simulink model "part1"  (R2021b)
settings: Solver=VariableStepAuto  StartTime=0.0  StopTime=t_set  MaxStep=dt  RelTol=1e-3
model workspace (MAT data in the model file):
  Amp = 1
values from neighbouring files (symbols this model uses):
  E = Vc(2)    [CurrentVelocities.m]
  Kd = [kd_surge kd_sway kd_yaw]    [CurrentVelocities.m]    (also in Init.m = [7e6 7e6 1e9])
  Ki = [ki_surge ki_sway ki_yaw]    [CurrentVelocities.m]    (also in Init.m = [3e6 3e6 1e6])
  Kp = [kp_surge kp_sway kp_yaw]    [CurrentVelocities.m]    (also in Init.m = [4e7 4e7 2e8])
  N = Vc(1)    [CurrentVelocities.m]
  set_x = 10    [CurrentVelocities.m]
  set_y = 10    [CurrentVelocities.m]
  set_yaw = 0.785    [CurrentVelocities.m]
  vessel =     [matlab.mat]
undefined symbols (not defined in the file or in its folder): Hoerner
libraries: marine_hydro x1
settings Model: Creator=jonbjor  LastModifiedBy=petterhangerhagen
settings SolverCC: AlgebraicLoopSolver=TrustRegion
settings DataIOCC: ReturnWorkspaceOutputs=off
settings DebuggingCC: SFMachineParentedDataDiag=warning  ArithmeticOperatorsInVariantConditions=warning
settings SFSimCC: SimUseLocalCustomCode=off  CustomCodeUndefinedFunction=UseInterfaceOnly
settings RTWCC: RTWUseLocalCustomCode=off

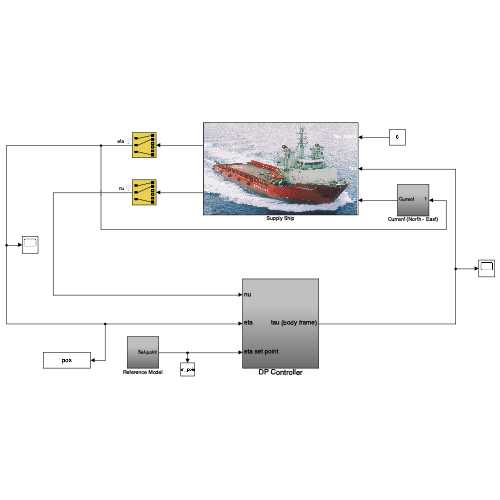
[thumbnail: Simulink's stored preview of the top-level diagram]
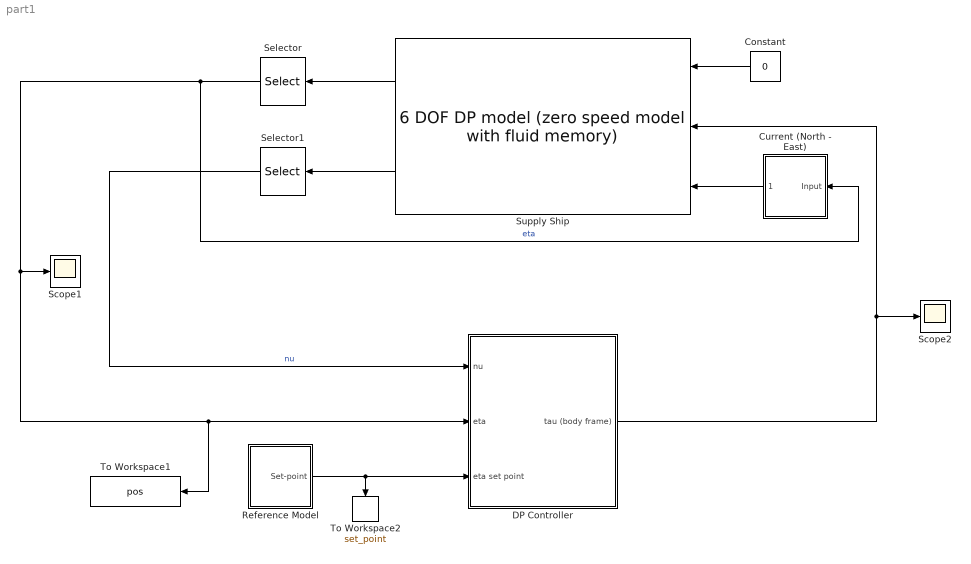
== system part1 ==
  Constant : Constant  Value=0
  Current (North - East) : Subsystem
  DP Controller : Subsystem
  Reference Model : Subsystem
  Scope1 : Scope
  Scope2 : Scope
  Selector : Selector  InputPortWidth=6  IndexOptions=Index vector (dialog)  Indices=[1 2 6]  OutputSizes=1
  Selector1 : Selector  InputPortWidth=6  IndexOptions=Index vector (dialog)  Indices=[1 2 6]  OutputSizes=1
  Supply Ship : marine_hydro/Hydro Library/6 DOF DP model  (zero speed model with fluid memory)  ABC=vesselABC  rho=1025  Axc=0.9*vessel.main.T*vessel.main.B  Ayc=0.9*vessel.main.T*vessel.main.Lpp  CX=1  CY_2D=Hoerner(vessel.main.B,vessel.main.T)  Bv=vessel.Bv  mask(6 DOF zero speed model){}
      link override "Integrator1 ": InitialCondition=nu0
      link override Integrator2: InitialCondition=eta0
      settings: SourceProductName=MSS Hydro
      mask Display:
      | image('supply.jpg');
      | color('white'); port_label('output', 1, 'eta')
      | color('white'); port_label('output', 2, 'nu')
      | color('white'); port_label('input', 1, 'tau_wave')
      | color('white'); port_label('input', 2, 'tau')
      | color('white'); port_label('input', 3, 'nu_c')
  To Workspace1 : ToWorkspace  VariableName=pos  SaveFormat=Timeseries  SampleTime=-1
  To Workspace2 : ToWorkspace  VariableName=set_point  SaveFormat=Timeseries  SampleTime=-1
  wires:
  Current (North - East)/1(Current) -> Supply Ship/3
  DP Controller/1(tau (body frame)) -> Scope2/1, Supply Ship/2
  Supply Ship/1 -> Selector/1
  Supply Ship/2 -> Selector1/1
  Selector/1 -> Current (North - East)/1(Input), Scope1/1, To Workspace1/1, DP Controller/2(eta)  "eta"
  Selector1/1 -> DP Controller/1(nu)  "nu"
  Constant/1 -> Supply Ship/1
  Reference Model/1(Set-point) -> To Workspace2/1, DP Controller/3(eta set point)

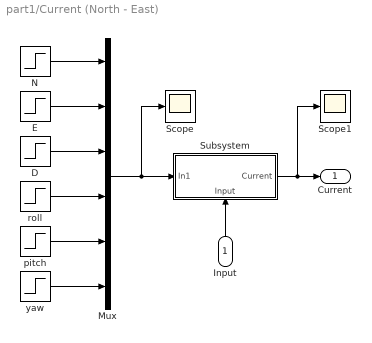
== system part1/Current (North - East) ==
  Input : Inport
  D : Step  Time=0  After=0  SampleTime=0
  E : Step  Time=0  After=E  SampleTime=0
  Mux : Mux  Inputs=6
  N : Step  Time=0  After=N  SampleTime=0
  Scope : Scope
  Scope1 : Scope
  Subsystem : Subsystem
      settings: PortSchema="{\"entries\":[{\"content\":{\"sides\":[{\"content\":{\"connectorIds\":[\"In1\"]},\"type\":\"ConnectorPlacement.EquallySpacedRectSide\",\"uuid\":\"4d23d725-1b89-4977-94a9-3d97af601562\"},{\"content\":{\"connectorIds\":[\"Out1\"],\"side\":\"RIGHT\"},\"type\":\"ConnectorPlacement.EquallySpacedRectSide\",\"uuid\":\"94064928-05d0-478d-b52c-d2c8e4fe82f6\"},{\"content\":{\"connectorIds\":[],\"side\":\"TOP\"},\"type\":\"ConnectorPlacement.EquallySpacedRectSide\",\"uuid\":\"63d93692-235d-465a-b22d-7c64b02cee26\"},{\"content\":{\"connectorIds\":[\"In2\"],\"side\":\"BOTTOM\"},\"type\":\"ConnectorPlacement.EquallySpacedRectSide\",\"uuid\":\"06906032-5717-4b79-be44-ac1ec3d34a3d\"}]},\"type\":\"ConnectorPlacement.EquallySpacedConnector\",\"uuid\":\"ca7e06dd-65f9-4f1a-a07c-a11377be80e1\"}],\"packageUris\":[\"http://schema.mathworks.com/mf0/Connector/R2020b\"],\"version\":\"1.0\"}"
  pitch : Step  Time=0  After=0  SampleTime=0
  roll : Step  Time=0  After=0  SampleTime=0
  yaw : Step  Time=0  After=0  SampleTime=0
  Current : Outport  VectorParamsAs1DForOutWhenUnconnected=off
  wires:
  N/1 -> Mux/1
  E/1 -> Mux/2
  Mux/1 -> Subsystem/1(In1), Scope/1
  D/1 -> Mux/3
  roll/1 -> Mux/4
  pitch/1 -> Mux/5
  yaw/1 -> Mux/6
  Input/1 -> Subsystem/2(Input)
  Subsystem/1(Current) -> Scope1/1, Current/1

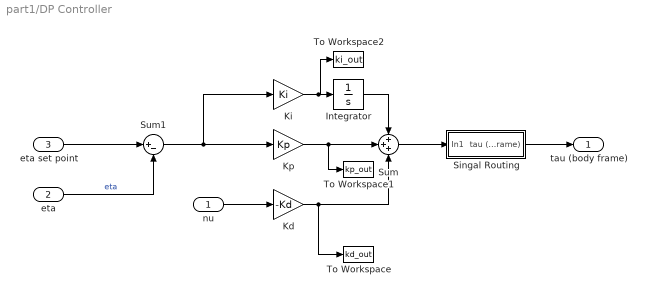
== system part1/DP Controller ==
  nu : Inport
  eta : Inport  Port=2
  eta set point : Inport  Port=3
  Integrator : Integrator
  Kd : Gain  Gain=-Kd
  Ki : Gain  Gain=Ki
  Kp : Gain  Gain=Kp
  Singal Routing : Subsystem
  Sum : Sum  Inputs=+++
  Sum1 : Sum  Inputs=|+-
  To Workspace : ToWorkspace  VariableName=kd_out  SaveFormat=Timeseries  SampleTime=-1
  To Workspace1 : ToWorkspace  VariableName=kp_out  SaveFormat=Timeseries  SampleTime=-1
  To Workspace2 : ToWorkspace  VariableName=ki_out  SaveFormat=Timeseries  SampleTime=-1
  tau (body frame) : Outport  VectorParamsAs1DForOutWhenUnconnected=off
  wires:
  Sum1/1 -> Ki/1, Kp/1
  eta set point/1 -> Sum1/1
  eta/1 -> Sum1/2  "eta"
  Kp/1 -> To Workspace1/1, Sum/2
  Ki/1 -> To Workspace2/1, Integrator/1
  Integrator/1 -> Sum/1
  Sum/1 -> Singal Routing/1(In1)
  Singal Routing/1(tau (body frame)) -> tau (body frame)/1
  Kd/1 -> Sum/3, To Workspace/1
  nu/1 -> Kd/1

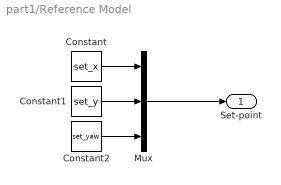
== system part1/Reference Model ==
  Constant : Constant  Value=set_x
  Constant1 : Constant  Value=set_y
  Constant2 : Constant  Value=set_yaw
  Mux : Mux  Inputs=3
  Set-point : Outport  VectorParamsAs1DForOutWhenUnconnected=off
  wires:
  Mux/1 -> Set-point/1
  Constant/1 -> Mux/1
  Constant1/1 -> Mux/2
  Constant2/1 -> Mux/3

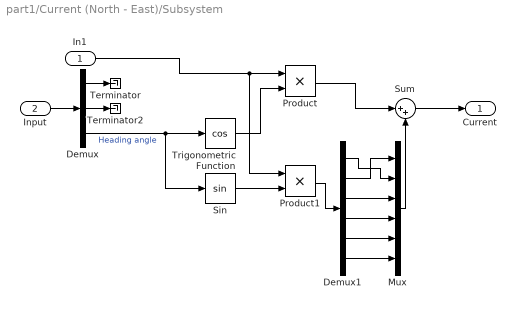
== system part1/Current (North - East)/Subsystem ==
  In1 : Inport
  Input : Inport  Port=2
  Demux : Demux  Outputs=3
  Demux1 : Demux  Outputs=6
  Mux : Mux  Inputs=6
  Product : Product
  Product1 : Product
  Sin : Trigonometry
  Sum : Sum  Inputs=|++
  Terminator : Terminator
  Terminator2 : Terminator
  Trigonometric Function : Trigonometry  Operator=cos
  Current : Outport
  wires:
  In1/1 -> Product1/1, Product/1
  Trigonometric Function/1 -> Product/2
  Demux/3 -> Sin/1, Trigonometric Function/1  "Heading angle"
  Input/1 -> Demux/1
  Demux/1 -> Terminator/1
  Demux/2 -> Terminator2/1
  Sin/1 -> Product1/2
  Product/1 -> Sum/1
  Sum/1 -> Current/1
  Product1/1 -> Demux1/1
  Demux1/2 -> Mux/1
  Demux1/1 -> Mux/2
  Demux1/3 -> Mux/3
  Demux1/4 -> Mux/4
  Demux1/5 -> Mux/5
  Demux1/6 -> Mux/6
  Mux/1 -> Sum/2

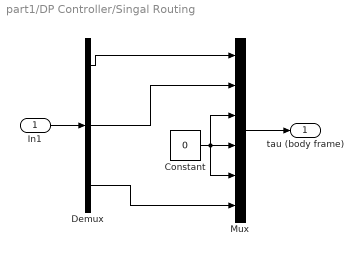
== system part1/DP Controller/Singal Routing ==
  In1 : Inport
  Constant : Constant  Value=0
  Demux : Demux  Outputs=3
  Mux : Mux  Inputs=6
  tau (body frame) : Outport
  wires:
  Demux/1 -> Mux/1
  Constant/1 -> Mux/5, Mux/3, Mux/4
  Demux/3 -> Mux/6
  In1/1 -> Demux/1
  Demux/2 -> Mux/2
  Mux/1 -> tau (body frame)/1
